simulink model "TestBench_DSD"  (R2021a)
settings: Solver=VariableStepAuto  StartTime=0.0  StopTime=0.05  FixedStep=1e-10  MaxStep=1e-4  RelTol=1e-3
PreLoadFcn:
  | clear;
  | dead_time= 5e-7;
  | T_sample = 1e-7;
  | f_pwm= 8e3;
  | f_el=200;
  | amplitude=0.1;
  | U_dc=800;
  | Iq_soll=200;
  | 
  | load('busdef.mat')
  | 
  | %**** Controller ****
  | L_filter = 70e-6;
  | R_losses = 1.74e-3;
  | PGain = L_filter*0.05*2*pi;
  | IGain = R_losses*0.05*2*pi;
  | 
  | %**** Deadtime Correction ****
  | Rds_on_module = 0.045/15;
  | 
  | %**** Filter ****
  | FilterQuality = 0.7071
InitFcn:
  | %%PGain = (L_filter*0.09*2*pi*f_pwm-R_losses)*0.45;
  | %%IGain = PGain*50/1.2; %% 25 = Period for ringing with too hight PGain
  | 
  | %%PGain = L_filter/(2*(1.5/f_pwm));
  | %%IGain  = PGain*R_losses/L_filter;
undefined symbols (not defined in the file): DiscIntNeverNeededParam, haltPwmSi, haltPwmSic, I_abc_sampled
libraries: nesl_utility x18, simulink x17, fl_lib x15, ee_lib x5, spsFirstOrderFilterLib x3, eeTransforms x2, cstextras x1, spsRMSLib x1, simulink_extras x1, spspowerguiLib x1
(part 2 of 3)

== system TestBench_DSD/Controller/Function-Call Subsystem4 ==
  function : TriggerPort  VariantControl=(inherit)
  Constant : Constant  Commented=on  Value=inf
  Constant1 : Constant  Commented=on
  Constant2 : Constant  Value=2
  Constant7 : Constant
  Data Store Read4 : DataStoreRead  DataStoreName=Inverter  IndexOptions=Index vector (dialog)  Indices=1  OutputSizes=1
  Data Store Write : DataStoreWrite  Commented=on  DataStoreName=Sic_PhU_ChB_On  IndexOptions=Index vector (dialog)  Indices=1  OutputSizes=1
  Data Store Write1 : DataStoreWrite  Commented=on  DataStoreName=Si_PhU_ChB_On  IndexOptions=Index vector (dialog)  Indices=1  OutputSizes=1
  Data Store Write2 : DataStoreWrite  DataStoreName=Inverter  IndexOptions=Index vector (dialog)  Indices=1  OutputSizes=1
  Data Store Write6 : DataStoreWrite  DataStoreName=haltPwmSi  DataStoreElements=haltPwmSi(2)  IndexOptions=Index vector (dialog)  Indices=1  OutputSizes=1
  MATLAB Function : MATLAB Function  TreatAsAtomicUnit=on
  wires:
  Constant/1 -> Data Store Write/1
  Constant1/1 -> Data Store Write1/1
  Constant7/1 -> Data Store Write6/1
  MATLAB Function/1(y) -> Data Store Write2/1
  Data Store Read4/1 -> MATLAB Function/2(devBus)
  Constant2/1 -> MATLAB Function/1(phase)

== system TestBench_DSD/Controller/Function-Call Subsystem5 ==
  function : TriggerPort  VariantControl=(inherit)
  Constant : Constant  Commented=on  Value=0
  Constant1 : Constant  Commented=on
  Constant2 : Constant  Commented=on  Value=0
  Constant3 : Constant  Commented=on  Value=-1
  Constant4 : Constant  Commented=on
  Constant5 : Constant  Commented=on
  Constant6 : Constant  Value=0
  Constant7 : Constant  Value=2
  Data Store Read4 : DataStoreRead  DataStoreName=Inverter  IndexOptions=Index vector (dialog)  Indices=1  OutputSizes=1
  Data Store Write : DataStoreWrite  Commented=on  DataStoreName=Sic_PhU_ChA_Off  IndexOptions=Index vector (dialog)  Indices=1  OutputSizes=1
  Data Store Write1 : DataStoreWrite  Commented=on  DataStoreName=Si_PhU_ChB_Off  IndexOptions=Index vector (dialog)  Indices=1  OutputSizes=1
  Data Store Write2 : DataStoreWrite  Commented=on  DataStoreName=Sic_PhU_ChA_On  IndexOptions=Index vector (dialog)  Indices=1  OutputSizes=1
  Data Store Write3 : DataStoreWrite  Commented=on  DataStoreName=Sic_PhU_ChB_Off  IndexOptions=Index vector (dialog)  Indices=1  OutputSizes=1
  Data Store Write4 : DataStoreWrite  Commented=on  DataStoreName=Si_PhU_ChA_Off  IndexOptions=Index vector (dialog)  Indices=1  OutputSizes=1
  Data Store Write5 : DataStoreWrite  Commented=on  DataStoreName=Si_PhU_ChA_On  IndexOptions=Index vector (dialog)  Indices=1  OutputSizes=1
  Data Store Write6 : DataStoreWrite  DataStoreName=Inverter  IndexOptions=Index vector (dialog)  Indices=1  OutputSizes=1
  Data Store Write7 : DataStoreWrite  DataStoreName=haltPwmSic  DataStoreElements=haltPwmSic(2)  IndexOptions=Index vector (dialog)  Indices=1  OutputSizes=1
  MATLAB Function : MATLAB Function  TreatAsAtomicUnit=on
  wires:
  Constant1/1 -> Data Store Write1/1
  Constant/1 -> Data Store Write/1
  Constant2/1 -> Data Store Write2/1
  Constant3/1 -> Data Store Write3/1
  Constant4/1 -> Data Store Write4/1
  Constant5/1 -> Data Store Write5/1
  Constant6/1 -> Data Store Write7/1
  MATLAB Function/1(y) -> Data Store Write6/1
  Data Store Read4/1 -> MATLAB Function/2(devBus)
  Constant7/1 -> MATLAB Function/1(phase)

== system TestBench_DSD/Controller/Function-Call Subsystem6 ==
  function : TriggerPort  VariantControl=(inherit)
  Constant : Constant  Commented=on
  Constant1 : Constant  Commented=on  Value=1e3
  Constant2 : Constant  Value=2
  Constant6 : Constant
  Data Store Read4 : DataStoreRead  DataStoreName=Inverter  IndexOptions=Index vector (dialog)  Indices=1  OutputSizes=1
  Data Store Write : DataStoreWrite  Commented=on  DataStoreName=Sic_PhU_ChB_On  IndexOptions=Index vector (dialog)  Indices=1  OutputSizes=1
  Data Store Write1 : DataStoreWrite  Commented=on  DataStoreName=Si_PhU_ChB_On  IndexOptions=Index vector (dialog)  Indices=1  OutputSizes=1
  Data Store Write2 : DataStoreWrite  DataStoreName=Inverter  IndexOptions=Index vector (dialog)  Indices=1  OutputSizes=1
  Data Store Write7 : DataStoreWrite  DataStoreName=haltPwmSic  DataStoreElements=haltPwmSic(2)  IndexOptions=Index vector (dialog)  Indices=1  OutputSizes=1
  MATLAB Function : MATLAB Function  TreatAsAtomicUnit=on
  wires:
  Constant/1 -> Data Store Write/1
  Constant1/1 -> Data Store Write1/1
  Constant6/1 -> Data Store Write7/1
  MATLAB Function/1(y) -> Data Store Write2/1
  Data Store Read4/1 -> MATLAB Function/2(devBus)
  Constant2/1 -> MATLAB Function/1(phase)

== system TestBench_DSD/Controller/Function-Call Subsystem7 ==
  function : TriggerPort  VariantControl=(inherit)
  Constant : Constant  Commented=on
  Constant1 : Constant  Commented=on  Value=-1
  Constant2 : Constant  Commented=on
  Constant3 : Constant  Commented=on
  Constant4 : Constant  Commented=on  Value=0
  Constant5 : Constant  Commented=on  Value=0
  Constant6 : Constant  Value=2
  Constant7 : Constant  Value=0
  Data Store Read4 : DataStoreRead  DataStoreName=Inverter  IndexOptions=Index vector (dialog)  Indices=1  OutputSizes=1
  Data Store Write : DataStoreWrite  Commented=on  DataStoreName=Sic_PhU_ChA_Off  IndexOptions=Index vector (dialog)  Indices=1  OutputSizes=1
  Data Store Write1 : DataStoreWrite  Commented=on  DataStoreName=Si_PhU_ChB_Off  IndexOptions=Index vector (dialog)  Indices=1  OutputSizes=1
  Data Store Write2 : DataStoreWrite  Commented=on  DataStoreName=Sic_PhU_ChA_On  IndexOptions=Index vector (dialog)  Indices=1  OutputSizes=1
  Data Store Write3 : DataStoreWrite  Commented=on  DataStoreName=Sic_PhU_ChB_Off  IndexOptions=Index vector (dialog)  Indices=1  OutputSizes=1
  Data Store Write4 : DataStoreWrite  Commented=on  DataStoreName=Si_PhU_ChA_Off  IndexOptions=Index vector (dialog)  Indices=1  OutputSizes=1
  Data Store Write5 : DataStoreWrite  Commented=on  DataStoreName=Si_PhU_ChA_On  IndexOptions=Index vector (dialog)  Indices=1  OutputSizes=1
  Data Store Write6 : DataStoreWrite  DataStoreName=haltPwmSi  DataStoreElements=haltPwmSi(2)  IndexOptions=Index vector (dialog)  Indices=1  OutputSizes=1
  Data Store Write7 : DataStoreWrite  DataStoreName=Inverter  IndexOptions=Index vector (dialog)  Indices=1  OutputSizes=1
  MATLAB Function : MATLAB Function  TreatAsAtomicUnit=on
  wires:
  Constant1/1 -> Data Store Write1/1
  Constant/1 -> Data Store Write/1
  Constant2/1 -> Data Store Write2/1
  Constant3/1 -> Data Store Write3/1
  Constant4/1 -> Data Store Write4/1
  Constant5/1 -> Data Store Write5/1
  Constant7/1 -> Data Store Write6/1
  Data Store Read4/1 -> MATLAB Function/2(devBus)
  MATLAB Function/1(y) -> Data Store Write7/1
  Constant6/1 -> MATLAB Function/1(phase)

== system TestBench_DSD/Controller/Function-Call Subsystem8 ==
  function : TriggerPort  VariantControl=(inherit)
  Constant : Constant  Commented=on  Value=inf
  Constant1 : Constant  Commented=on
  Constant2 : Constant  Value=3
  Constant7 : Constant
  Data Store Read4 : DataStoreRead  DataStoreName=Inverter  IndexOptions=Index vector (dialog)  Indices=1  OutputSizes=1
  Data Store Write : DataStoreWrite  Commented=on  DataStoreName=Sic_PhU_ChB_On  IndexOptions=Index vector (dialog)  Indices=1  OutputSizes=1
  Data Store Write1 : DataStoreWrite  Commented=on  DataStoreName=Si_PhU_ChB_On  IndexOptions=Index vector (dialog)  Indices=1  OutputSizes=1
  Data Store Write2 : DataStoreWrite  DataStoreName=Inverter  IndexOptions=Index vector (dialog)  Indices=1  OutputSizes=1
  Data Store Write6 : DataStoreWrite  DataStoreName=haltPwmSi  DataStoreElements=haltPwmSi(3)  IndexOptions=Index vector (dialog)  Indices=1  OutputSizes=1
  MATLAB Function : MATLAB Function  TreatAsAtomicUnit=on
  wires:
  Constant/1 -> Data Store Write/1
  Constant1/1 -> Data Store Write1/1
  Constant7/1 -> Data Store Write6/1
  MATLAB Function/1(y) -> Data Store Write2/1
  Data Store Read4/1 -> MATLAB Function/2(devBus)
  Constant2/1 -> MATLAB Function/1(phase)

== system TestBench_DSD/Controller/Function-Call Subsystem9 ==
  function : TriggerPort  VariantControl=(inherit)
  Constant : Constant  Commented=on  Value=0
  Constant1 : Constant  Commented=on
  Constant2 : Constant  Commented=on  Value=0
  Constant3 : Constant  Commented=on  Value=-1
  Constant4 : Constant  Commented=on
  Constant5 : Constant  Commented=on
  Constant6 : Constant  Value=0
  Constant7 : Constant  Value=3
  Data Store Read4 : DataStoreRead  DataStoreName=Inverter  IndexOptions=Index vector (dialog)  Indices=1  OutputSizes=1
  Data Store Write : DataStoreWrite  Commented=on  DataStoreName=Sic_PhU_ChA_Off  IndexOptions=Index vector (dialog)  Indices=1  OutputSizes=1
  Data Store Write1 : DataStoreWrite  Commented=on  DataStoreName=Si_PhU_ChB_Off  IndexOptions=Index vector (dialog)  Indices=1  OutputSizes=1
  Data Store Write2 : DataStoreWrite  Commented=on  DataStoreName=Sic_PhU_ChA_On  IndexOptions=Index vector (dialog)  Indices=1  OutputSizes=1
  Data Store Write3 : DataStoreWrite  Commented=on  DataStoreName=Sic_PhU_ChB_Off  IndexOptions=Index vector (dialog)  Indices=1  OutputSizes=1
  Data Store Write4 : DataStoreWrite  Commented=on  DataStoreName=Si_PhU_ChA_Off  IndexOptions=Index vector (dialog)  Indices=1  OutputSizes=1
  Data Store Write5 : DataStoreWrite  Commented=on  DataStoreName=Si_PhU_ChA_On  IndexOptions=Index vector (dialog)  Indices=1  OutputSizes=1
  Data Store Write6 : DataStoreWrite  DataStoreName=Inverter  IndexOptions=Index vector (dialog)  Indices=1  OutputSizes=1
  Data Store Write7 : DataStoreWrite  DataStoreName=haltPwmSic  DataStoreElements=haltPwmSic(3)  IndexOptions=Index vector (dialog)  Indices=1  OutputSizes=1
  MATLAB Function : MATLAB Function  TreatAsAtomicUnit=on
  wires:
  Constant1/1 -> Data Store Write1/1
  Constant/1 -> Data Store Write/1
  Constant2/1 -> Data Store Write2/1
  Constant3/1 -> Data Store Write3/1
  Constant4/1 -> Data Store Write4/1
  Constant5/1 -> Data Store Write5/1
  Constant6/1 -> Data Store Write7/1
  MATLAB Function/1(y) -> Data Store Write6/1
  Data Store Read4/1 -> MATLAB Function/2(devBus)
  Constant7/1 -> MATLAB Function/1(phase)

== system TestBench_DSD/Controller/Subsystem ==
  u : Inport
  cutoff frequency : Inport  Port=2
  Constant : Constant  Value=f_pwm
  MATLAB Function : cstextras/DiscreteFirstOrderSection/MATLAB Function  Tag=#GainSurfaceTarget_  SystemSampleTime=-1  VariantActivationTime=update diagram  Latency=0  AutoFrameSizeCalculation=off
      settings: SourceProductBaseCode=CT
  MATLAB Function1 : MATLAB Function  TreatAsAtomicUnit=on
  Product1 : Product
  Product4 : Product
  Sum : Sum  Inputs=|++
  Sum3 : Sum  Inputs=+|+
  Unit Delay : UnitDelay  SampleTime=-1  HasFrameUpgradeWarning=on
  y : Outport  VectorParamsAs1DForOutWhenUnconnected=off
  wires:
  u/1 -> Sum/1, Sum3/1
  Sum/1 -> Product1/2, Product4/2
  Product4/1 -> Sum3/2
  Sum3/1 -> Unit Delay/1
  cutoff frequency/1 -> MATLAB Function1/1(fc), MATLAB Function/1
  Unit Delay/1 -> Sum/2
  MATLAB Function/2 -> Product4/1
  MATLAB Function/1 -> Product1/1
  Product1/1 -> y/1
  MATLAB Function1/1(tau) -> MATLAB Function/2
  Constant/1 -> MATLAB Function1/2(fpwm)

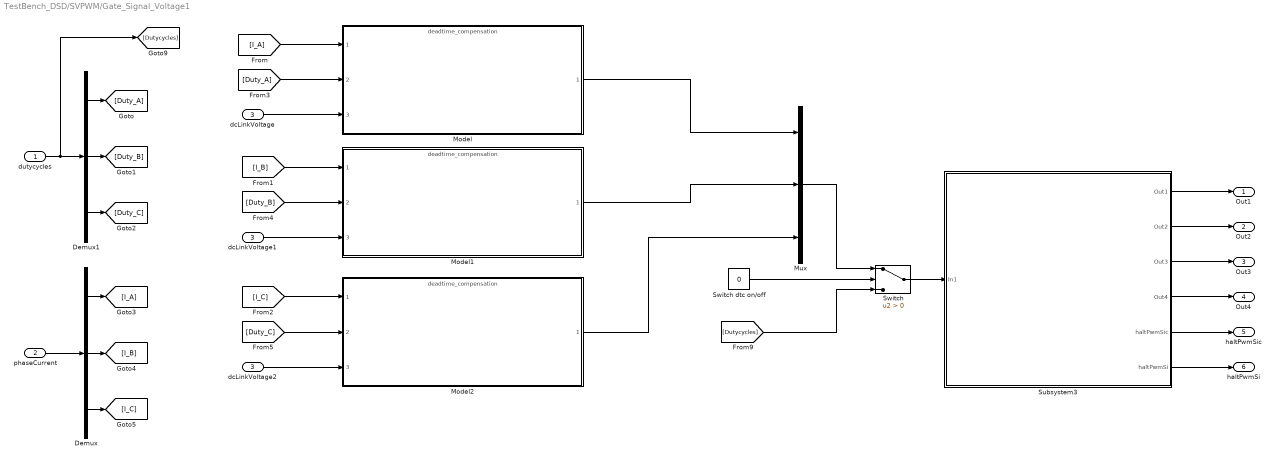
== system TestBench_DSD/SVPWM/Gate_Signal_Voltage1 ==
  dutycycles : Inport
  phaseCurrent : Inport  Port=2
  dcLinkVoltage : Inport  Port=3
  Demux : Demux  Outputs=3
  Demux1 : Demux  Outputs=3
  Model : ModelReference  ModelNameDialog=deadtime_compensation.slx  SimulationMode=Normal  ModelReferenceVersion=8.3
  Model1 : ModelReference  ModelNameDialog=deadtime_compensation.slx  SimulationMode=Normal  ModelReferenceVersion=8.3
  Model2 : ModelReference  ModelNameDialog=deadtime_compensation.slx  SimulationMode=Normal  ModelReferenceVersion=8.3
  Mux : Mux  Inputs=3
  Subsystem3 : Subsystem
  Switch : Switch  Criteria=u2 > Threshold
  Switch dtc on/off : Constant  Value=0
  dcLinkVoltage1 : InportShadow  Port=3
  dcLinkVoltage2 : InportShadow  Port=3
  Out1 : Outport
  Out2 : Outport  Port=2
  Out3 : Outport  Port=3
  Out4 : Outport  Port=4
  haltPwmSic : Outport  Port=5
  haltPwmSi : Outport  Port=6
  wires:
  phaseCurrent/1 -> Demux/1
  Demux1/1 -> [Duty_A]
  Demux1/2 -> [Duty_B]
  Demux1/3 -> [Duty_C]
  Demux/1 -> [I_A]
  Demux/2 -> [I_B]
  Demux/3 -> [I_C]
  [I_A] -> Model/1
  [Duty_A] -> Model/2
  Model/1 -> Mux/1
  [I_B] -> Model1/1
  [Duty_B] -> Model1/2
  Model1/1 -> Mux/2
  [Duty_C] -> Model2/2
  Switch dtc on/off/1 -> Switch/2
  [Dutycycles] -> Switch/3
  Mux/1 -> Switch/1
  dutycycles/1 -> Demux1/1, [Dutycycles]
  Model2/1 -> Mux/3
  Switch/1 -> Subsystem3/1(In1)
  Subsystem3/2(Out2) -> Out2/1
  Subsystem3/4(Out4) -> Out4/1
  Subsystem3/3(Out3) -> Out3/1
  Subsystem3/1(Out1) -> Out1/1
  Subsystem3/5(haltPwmSic) -> haltPwmSic/1
  Subsystem3/6(haltPwmSi) -> haltPwmSi/1
  [I_C] -> Model2/1
  dcLinkVoltage1/1 -> Model1/3
  dcLinkVoltage/1 -> Model/3
  dcLinkVoltage2/1 -> Model2/3

== system TestBench_DSD/SVPWM/SVPWM ==
  U_mag : Inport
  U_angle : Inport  Port=2
  Constant4 : Constant  Value=f_pwm
  Constant5 : Constant  Value=0
  Constant6 : Constant  Value=0
  Determine reference vector (U*) : Subsystem
  INFO : Subsystem
      mask Display: disp('?')
  SV Modulator Pattern #1 : Subsystem
  Sector Number : Outport  VectorParamsAs1DForOutWhenUnconnected=off
  Ta Tb T0 normalized : Outport  Port=2  VectorParamsAs1DForOutWhenUnconnected=off
  wires:
  SV Modulator Pattern #1/1(Sector Number) -> Sector Number/1
  SV Modulator Pattern #1/2(Ta Tb T0 normalized) -> Ta Tb T0 normalized/1
  U_angle/1 -> Determine reference vector (U*)/2(In2)
  Determine reference vector (U*)/2(alpha) -> SV Modulator Pattern #1/2(alpha)
  Constant6/1 -> Determine reference vector (U*)/5(Pha_Init)
  Determine reference vector (U*)/1(m) -> SV Modulator Pattern #1/1(m)
  Constant5/1 -> Determine reference vector (U*)/3(m_Int)
  Constant4/1 -> Determine reference vector (U*)/4(Freq_Int)
  U_mag/1 -> Determine reference vector (U*)/1(In1)

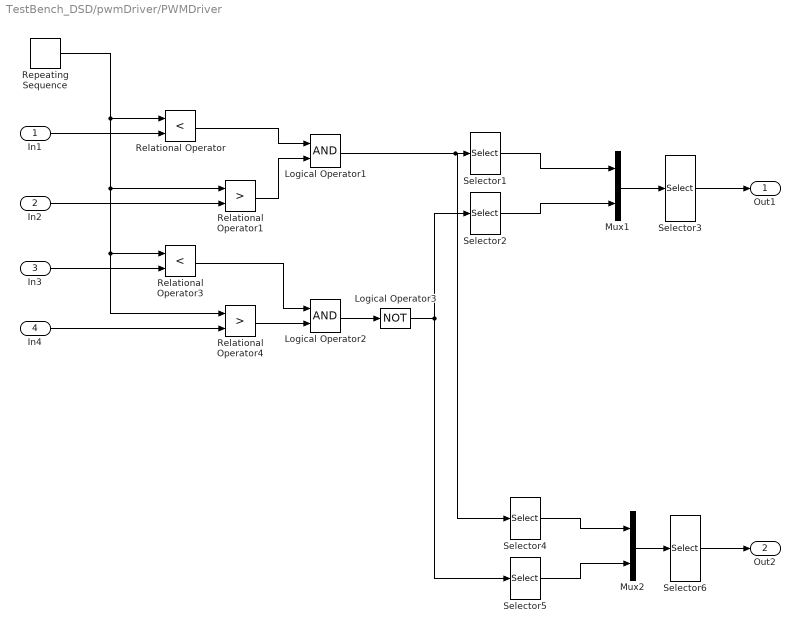
== system TestBench_DSD/pwmDriver/PWMDriver ==
  In1 : Inport
  In2 : Inport  Port=2
  In3 : Inport  Port=3
  In4 : Inport  Port=4
  Logical Operator1 : Logic  AllPortsSameDT=off  OutDataTypeStr=boolean
  Logical Operator2 : Logic  AllPortsSameDT=off  OutDataTypeStr=boolean
  Logical Operator3 : Logic  Operator=NOT  AllPortsSameDT=off  OutDataTypeStr=boolean
  Mux1 : Mux  Inputs=2
  Mux2 : Mux  Inputs=2
  Relational Operator : RelationalOperator  Operator=<  OutDataTypeStr=boolean  RndMeth=Simplest
  Relational Operator1 : RelationalOperator  Operator=>  OutDataTypeStr=boolean  RndMeth=Simplest
  Relational Operator3 : RelationalOperator  Operator=<  OutDataTypeStr=boolean  RndMeth=Simplest
  Relational Operator4 : RelationalOperator  Operator=>  OutDataTypeStr=boolean  RndMeth=Simplest
  Repeating Sequence : simulink/Sources/Repeating Sequence  rep_seq_t=[0 1/f_pwm]  rep_seq_y=[0 1/f_pwm]
  Selector1 : Selector  InputPortWidth=6  IndexOptions=Index vector (dialog)  Indices=[1 2 3]  OutputSizes=1
  Selector2 : Selector  InputPortWidth=6  IndexOptions=Index vector (dialog)  Indices=[1 2 3]  OutputSizes=1
  Selector3 : Selector  InputPortWidth=6  IndexOptions=Index vector (dialog)  Indices=[1 4 2 5 3 6]  OutputSizes=1
  Selector4 : Selector  InputPortWidth=6  IndexOptions=Index vector (dialog)  Indices=[4 5 6]  OutputSizes=1
  Selector5 : Selector  InputPortWidth=6  IndexOptions=Index vector (dialog)  Indices=[4 5 6]  OutputSizes=1
  Selector6 : Selector  InputPortWidth=6  IndexOptions=Index vector (dialog)  Indices=[1 4 2 5 3 6]  OutputSizes=1
  Out1 : Outport
  Out2 : Outport  Port=2
  wires:
  Repeating Sequence/1 -> Relational Operator/1, Relational Operator4/1, Relational Operator3/1, Relational Operator1/1
  Logical Operator1/1 -> Selector4/1, Selector1/1
  Mux1/1 -> Selector3/1
  Selector2/1 -> Mux1/2
  Mux2/1 -> Selector6/1
  Relational Operator3/1 -> Logical Operator2/1
  Logical Operator3/1 -> Selector5/1, Selector2/1
  Relational Operator4/1 -> Logical Operator2/2
  Logical Operator2/1 -> Logical Operator3/1
  In3/1 -> Relational Operator3/2
  Selector5/1 -> Mux2/2
  Relational Operator1/1 -> Logical Operator1/2
  Selector1/1 -> Mux1/1
  Relational Operator/1 -> Logical Operator1/1
  Selector4/1 -> Mux2/1
  Selector3/1 -> Out1/1
  Selector6/1 -> Out2/1
  In4/1 -> Relational Operator4/2
  In1/1 -> Relational Operator/2
  In2/1 -> Relational Operator1/2

== system TestBench_DSD/Controller/Discrete PI Controller Id/Clamping circuit ==
  preSat : Inport  DisableCoverage=on
  preIntegrator : Inport  DisableCoverage=on  Port=2
  AND : Logic  DisableCoverage=on
  Data Store Read1 : DataStoreRead  DataStoreName=dc_voltage_sampled  IndexOptions=Index vector (dialog)  Indices=1  OutputSizes=1
  Data Store Read5 : DataStoreRead  DataStoreName=dc_voltage_sampled  IndexOptions=Index vector (dialog)  Indices=1  OutputSizes=1
  DataTypeConv1 : DataTypeConversion  DisableCoverage=on  OutDataTypeStr=int8  SaturateOnIntegerOverflow=on  RndMeth=Zero  LockScale=on
  DataTypeConv2 : DataTypeConversion  DisableCoverage=on  OutDataTypeStr=int8
  Dead Zone Dynamic : simulink/Discontinuities/Dead Zone Dynamic
      settings: SourceProductBaseCode=SL
  Equal : RelationalOperator  DisableCoverage=on  Operator===  RndMeth=Nearest  InputSameDT=on
  Gain : Gain  Gain=-1
  NotEqual : RelationalOperator  DisableCoverage=on  Operator=~=  RndMeth=Nearest  InputSameDT=on
  SignDeltaU : Signum  DisableCoverage=on
  SignPreIntegrator : Signum  DisableCoverage=on
  ZeroGain : Gain  DisableCoverage=on  Gain=0  SaturateOnIntegerOverflow=on  OutDataTypeStr=Inherit: Same as input  ParamDataTypeStr=Inherit: Same as input
  Clamp : Outport  DisableCoverage=on  VectorParamsAs1DForOutWhenUnconnected=off
  wires:
  preSat/1 -> Dead Zone Dynamic/2, ZeroGain/1
  preIntegrator/1 -> SignPreIntegrator/1
  ZeroGain/1 -> NotEqual/1
  Dead Zone Dynamic/1 -> NotEqual/2, SignDeltaU/1
  SignDeltaU/1 -> DataTypeConv1/1
  DataTypeConv1/1 -> Equal/1
  SignPreIntegrator/1 -> DataTypeConv2/1
  DataTypeConv2/1 -> Equal/2
  NotEqual/1 -> AND/1
  Equal/1 -> AND/2
  AND/1 -> Clamp/1
  Data Store Read1/1 -> Gain/1
  Data Store Read5/1 -> Dead Zone Dynamic/1
  Gain/1 -> Dead Zone Dynamic/3

== system TestBench_DSD/Controller/Discrete PI Controller Iq/Clamping circuit ==
  preSat : Inport  DisableCoverage=on
  preIntegrator : Inport  DisableCoverage=on  Port=2
  AND : Logic  DisableCoverage=on
  Data Store Read1 : DataStoreRead  DataStoreName=dc_voltage_sampled  IndexOptions=Index vector (dialog)  Indices=1  OutputSizes=1
  Data Store Read5 : DataStoreRead  DataStoreName=dc_voltage_sampled  IndexOptions=Index vector (dialog)  Indices=1  OutputSizes=1
  DataTypeConv1 : DataTypeConversion  DisableCoverage=on  OutDataTypeStr=int8  SaturateOnIntegerOverflow=on  RndMeth=Zero  LockScale=on
  DataTypeConv2 : DataTypeConversion  DisableCoverage=on  OutDataTypeStr=int8
  Dead Zone Dynamic : simulink/Discontinuities/Dead Zone Dynamic
      settings: SourceProductBaseCode=SL
  Equal : RelationalOperator  DisableCoverage=on  Operator===  RndMeth=Nearest  InputSameDT=on
  Gain : Gain  Gain=-1
  NotEqual : RelationalOperator  DisableCoverage=on  Operator=~=  RndMeth=Nearest  InputSameDT=on
  SignDeltaU : Signum  DisableCoverage=on
  SignPreIntegrator : Signum  DisableCoverage=on
  ZeroGain : Gain  DisableCoverage=on  Gain=0  SaturateOnIntegerOverflow=on  OutDataTypeStr=Inherit: Same as input  ParamDataTypeStr=Inherit: Same as input
  Clamp : Outport  DisableCoverage=on  VectorParamsAs1DForOutWhenUnconnected=off
  wires:
  Gain/1 -> Dead Zone Dynamic/3
  Data Store Read5/1 -> Dead Zone Dynamic/1
  Data Store Read1/1 -> Gain/1
  AND/1 -> Clamp/1
  Equal/1 -> AND/2
  NotEqual/1 -> AND/1
  DataTypeConv2/1 -> Equal/2
  SignPreIntegrator/1 -> DataTypeConv2/1
  DataTypeConv1/1 -> Equal/1
  SignDeltaU/1 -> DataTypeConv1/1
  Dead Zone Dynamic/1 -> SignDeltaU/1, NotEqual/2
  ZeroGain/1 -> NotEqual/1
  preIntegrator/1 -> SignPreIntegrator/1
  preSat/1 -> ZeroGain/1, Dead Zone Dynamic/2

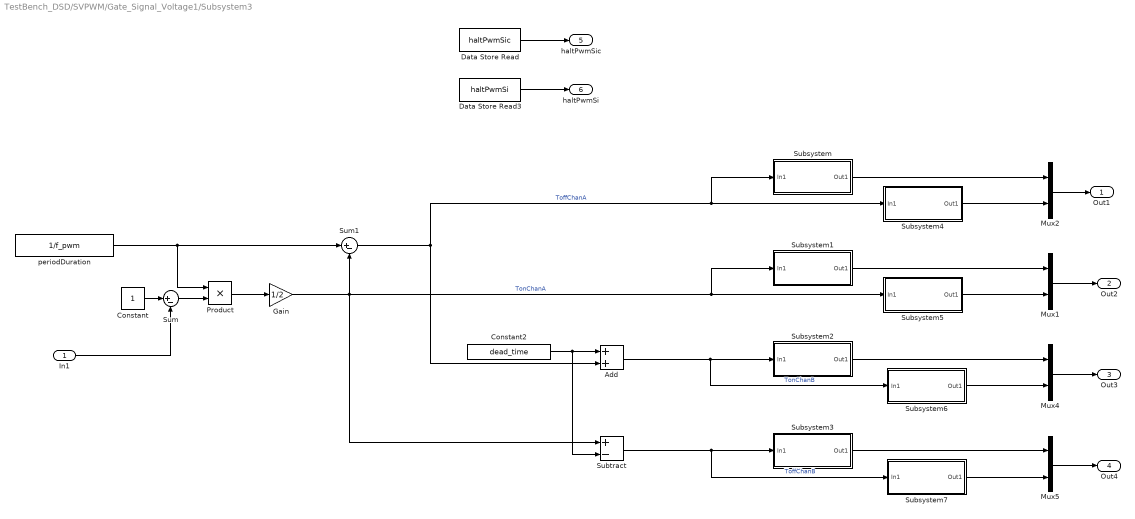
== system TestBench_DSD/SVPWM/Gate_Signal_Voltage1/Subsystem3 ==
  In1 : Inport
  Add : Sum
  Constant : Constant
  Constant2 : Constant  Value=dead_time
  Data Store Read : DataStoreRead  DataStoreName=haltPwmSic  IndexOptions=Index vector (dialog)  Indices=1  OutputSizes=1
  Data Store Read3 : DataStoreRead  DataStoreName=haltPwmSi  IndexOptions=Index vector (dialog)  Indices=1  OutputSizes=1
  Gain : Gain  Gain=1/2
  Mux{1..2,4..5} (4 alike) : Mux  Inputs=2
  Product : Product
  Subsystem : Subsystem
  Subsystem1 : Subsystem
  Subsystem2 : Subsystem
  Subsystem3 : Subsystem
  Subsystem4 : Subsystem
  Subsystem5 : Subsystem
  Subsystem6 : Subsystem
  Subsystem7 : Subsystem
  Subtract : Sum  Inputs=+-
  Sum : Sum  Inputs=|+-
  Sum1 : Sum  Inputs=|+-
  periodDuration : Constant  Value=1/f_pwm
  Out1 : Outport
  Out2 : Outport  Port=2
  Out3 : Outport  Port=3
  Out4 : Outport  Port=4
  haltPwmSic : Outport  Port=5
  haltPwmSi : Outport  Port=6
  wires:
  In1/1 -> Sum/2
  Constant2/1 -> Add/1, Subtract/2
  Sum1/1 -> Subsystem4/1(In1), Subsystem/1(In1), Add/2  "ToffChanA"
  periodDuration/1 -> Sum1/1, Product/1
  Gain/1 -> Subtract/1, Sum1/2, Subsystem5/1(In1), Subsystem1/1(In1)  "TonChanA"
  Constant/1 -> Sum/1
  Add/1 -> Subsystem2/1(In1), Subsystem6/1(In1)  "TonChanB"
  Product/1 -> Gain/1
  Mux2/1 -> Out1/1
  Subtract/1 -> Subsystem3/1(In1), Subsystem7/1(In1)  "ToffChanB"
  Mux4/1 -> Out3/1
  Sum/1 -> Product/2
  Mux5/1 -> Out4/1
  Mux1/1 -> Out2/1
  Subsystem/1(Out1) -> Mux2/1
  Subsystem1/1(Out1) -> Mux1/1
  Subsystem2/1(Out1) -> Mux4/1
  Subsystem3/1(Out1) -> Mux5/1
  Subsystem4/1(Out1) -> Mux2/2
  Subsystem5/1(Out1) -> Mux1/2
  Subsystem6/1(Out1) -> Mux4/2
  Subsystem7/1(Out1) -> Mux5/2
  Data Store Read/1 -> haltPwmSic/1
  Data Store Read3/1 -> haltPwmSi/1

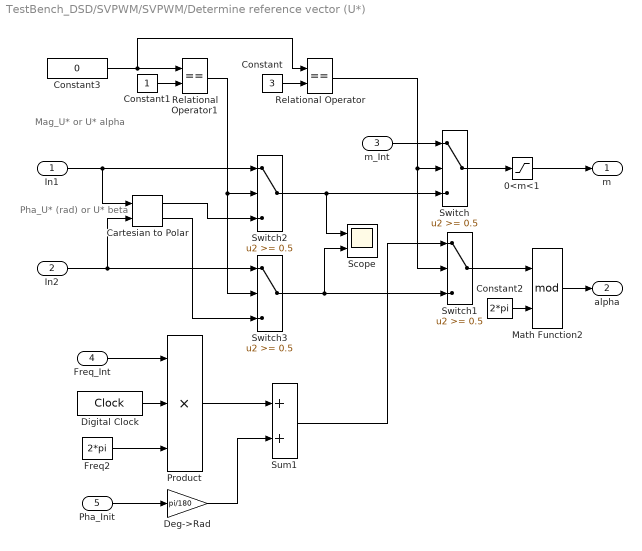
== system TestBench_DSD/SVPWM/SVPWM/Determine reference vector (U*) ==
  note: Pha_U* (rad)
      | or
      | U* beta
  note: Mag_U*
      | or
      | U* alpha
  In1 : Inport
  In2 : Inport  Port=2
  m_Int : Inport  Port=3
  Freq_Int : Inport  Port=4
  Pha_Init : Inport  Port=5
  "0<m<1 " : Saturate  UpperLimit=1  LowerLimit=0
  Cartesian to Polar : simulink_extras/Transformations/Cartesian to Polar
  Constant : Constant  Value=3
  Constant1 : Constant
  Constant2 : Constant  Value=2*pi
  Constant3 : Constant  Value=0
  Deg->Rad : Gain  Gain=pi/180  SaturateOnIntegerOverflow=on  OutDataTypeStr=Inherit: Same as input  ParamDataTypeStr=Inherit: Same as input
  Digital Clock : DigitalClock  SampleTime=-1
  Freq2 : Constant  Value=2*pi
  Math Function2 : Math  Operator=mod  SignedPower=on  SaturateOnIntegerOverflow=on
  Product : Product  Inputs=***  InputSameDT=on  SaturateOnIntegerOverflow=on  OutDataTypeStr=Inherit: Same as first input
  Relational Operator : RelationalOperator  Operator===  RndMeth=Nearest
  Relational Operator1 : RelationalOperator  Operator===  RndMeth=Nearest
  Scope : Scope  NumInputPorts=2
  Sum1 : Sum  InputSameDT=on  SaturateOnIntegerOverflow=on  OutDataTypeStr=Inherit: Same as first input
  Switch{,1..3} (4 alike) : Switch  Threshold=0.5  SaturateOnIntegerOverflow=on
  m : Outport  VectorParamsAs1DForOutWhenUnconnected=off
  alpha : Outport  Port=2  VectorParamsAs1DForOutWhenUnconnected=off
  wires:
  Digital Clock/1 -> Product/2
  Switch1/1 -> Math Function2/1
  Sum1/1 -> Switch1/1
  Math Function2/1 -> alpha/1
  Constant2/1 -> Math Function2/2
  Relational Operator1/1 -> Switch3/2, Switch2/2
  Cartesian to Polar/2 -> Switch3/3
  Cartesian to Polar/1 -> Switch2/3
  Switch2/1 -> Scope/1, Switch/3
  Constant3/1 -> Relational Operator/1, Relational Operator1/1
  Constant1/1 -> Relational Operator1/2
  Relational Operator/1 -> Switch/2, Switch1/2
  Constant/1 -> Relational Operator/2
  m_Int/1 -> Switch/1
  In2/1 -> Switch3/1, Cartesian to Polar/2
  In1/1 -> Switch2/1, Cartesian to Polar/1
  "0<m<1 "/1 -> m/1
  Switch/1 -> "0<m<1 "/1
  Freq2/1 -> Product/3
  Freq_Int/1 -> Product/1
  Deg->Rad/1 -> Sum1/2
  Pha_Init/1 -> Deg->Rad/1
  Product/1 -> Sum1/1
  Switch3/1 -> Scope/2, Switch1/3

== system TestBench_DSD/SVPWM/SVPWM/INFO ==
  note: Pattern #2:
      | With this pattern, identified as "Hardware-Determined" by Texas Instruments, there is always one PWM channel staying constant for the entire PWM period.
      |  So the number of switching times for this pattern is less than pattern #1. As a result, switching losses will be reduced with Pattern #2.
  note: Pattern #1:
      | With this pattern, identified as "Software-Determined" by Texas Instruments, each PWM channel switches twice per every PWM period.
  note: --------------------------------------------------------------------------------------------------------------------------------------------------------------------
  note: Reference: Application Report SPRA524
      | Space-Vector PWM with TMS320C24x Using H/W & S/W Determined Switching Patterns
      | Zhenyu Yu, Texas Instruments
  note: The objective of the SV PWM technique is to approximate the reference voltage vector (U*) instantaneously
      | by combination of the switching states corresponding to the basic space vectors.
  note: U7 = 1 1 1
  note: Q1 Q3 Q5
  note: --------------------------------------------------------
  note: Three-Phase VSC Diagram
  note: -
  note: +
  note: --------------------------------------------------------
  note: |
      | |
      | |
  note: ---Vc
  note: |
      | |
      | |
  note: |
      | |
      | |
      | |
      | |
      | |
  note: [Q6]
  note: [Q5]
  note: |
      | |
      | |
  note: ---Vb
  note: |
      | |
      | |
  note: |
      | |
      | |
      | |
      | |
      | |
  note: [Q4]
  note: [Q3]
  note: |
      | |
      | |
  note: ---Va
  note: |
      | |
      | |
  note: |
      | |
      | |
      | |
      | |
      | |
  note: [Q2]
  note: [Q1]
  note: Vdc
  note: [n] = Sector number
  note: [2]
  note: Basic Space Vectors and Switching States
  note: U4 = 0 1 1
  note: U5 = 0 0 1
  note: U6 = 1 0 1
  note: U0 = 0 0 0
  note: U3 = 0 1 0
  note: U2 = 1 1 0
  note: U1 = 1 0 0
  note: [6]
  note: [5]
  note: [4]
  note: [3]
  note: [1]
  note: 3                       2
      |       3                   2
      |         3               2
      |           3           2
      |             3       2
      |               3   2
      | 4 4 4 4 4 4 4 4 0 1 1 1 1 1 1 1 1
      |               5   6
      |             5       6
      |           5           6
      |         5               6
      |       5                   6
      |     5                       6
  note: Two symmetrical switching patterns have been implemented:

== system TestBench_DSD/SVPWM/SVPWM/SV Modulator Pattern #1 ==
  m : Inport
  alpha : Inport  Port=2
  "Compute time duration of switching states (Ta,Tb,To) " : Subsystem
  "Determine the sector of U* based on alpha (rad). Also, determine if the sector number is odd" : Subsystem
  INFO : Subsystem
      mask Display: disp('?')
  Sector Number : Outport  VectorParamsAs1DForOutWhenUnconnected=off
  Ta Tb T0 normalized : Outport  Port=2  VectorParamsAs1DForOutWhenUnconnected=off
  wires:
  m/1 -> "Compute time duration of switching states (Ta,Tb,To) "/2(m)
  alpha/1 -> "Compute time duration of switching states (Ta,Tb,To) "/1(alpha), "Determine the sector of U* based on alpha (rad). Also, determine if the sector number is odd"/1(alpha)
  "Compute time duration of switching states (Ta,Tb,To) "/1(Ta Tb T0 normalized) -> Ta Tb T0 normalized/1
  "Determine the sector of U* based on alpha (rad). Also, determine if the sector number is odd"/2(Odd_S) -> "Compute time duration of switching states (Ta,Tb,To) "/4(Odd_S)
  "Determine the sector of U* based on alpha (rad). Also, determine if the sector number is odd"/1(Sn) -> Sector Number/1, "Compute time duration of switching states (Ta,Tb,To) "/3(Sn)

== system TestBench_DSD/SVPWM/Gate_Signal_Voltage1/Subsystem3/Subsystem ==
  In1 : Inport
  Data Store Read2 : DataStoreRead  DataStoreName=Inverter  DataStoreElements=Inverter.V.Sic.ChA.TOn.enable  IndexOptions=Index vector (dialog)  Indices=1  OutputSizes=1
  Data Store Read4 : DataStoreRead  DataStoreName=Inverter  DataStoreElements=Inverter.U.Sic.ChA.TOn.enable  IndexOptions=Index vector (dialog)  Indices=1  OutputSizes=1
  Data Store Read5 : DataStoreRead  DataStoreName=Inverter  DataStoreElements=Inverter.W.Sic.ChA.TOn.enable  IndexOptions=Index vector (dialog)  Indices=1  OutputSizes=1
  Demux : Demux  Outputs=3
  Mux : Mux  Inputs=3
  Product : Product
  Product1 : Product
  Product2 : Product
  Out1 : Outport
  wires:
  In1/1 -> Demux/1
  Data Store Read4/1 -> Product/1
  Demux/1 -> Product/2
  Demux/2 -> Product1/2
  Demux/3 -> Product2/2
  Data Store Read5/1 -> Product2/1
  Data Store Read2/1 -> Product1/1
  Product1/1 -> Mux/2
  Mux/1 -> Out1/1
  Product2/1 -> Mux/3
  Product/1 -> Mux/1

== system TestBench_DSD/SVPWM/Gate_Signal_Voltage1/Subsystem3/Subsystem1 ==
  In1 : Inport
  Data Store Read : DataStoreRead  DataStoreName=Inverter  DataStoreElements=Inverter.U.Sic.ChA.TOff.enable  IndexOptions=Index vector (dialog)  Indices=1  OutputSizes=1
  Data Store Read1 : DataStoreRead  DataStoreName=Inverter  DataStoreElements=Inverter.V.Sic.ChA.TOff.enable  IndexOptions=Index vector (dialog)  Indices=1  OutputSizes=1
  Data Store Read3 : DataStoreRead  DataStoreName=Inverter  DataStoreElements=Inverter.W.Sic.ChA.TOff.enable  IndexOptions=Index vector (dialog)  Indices=1  OutputSizes=1
  Demux : Demux  Outputs=3
  Mux : Mux  Inputs=3
  Product : Product
  Product1 : Product
  Product2 : Product
  Out1 : Outport
  wires:
  Product/1 -> Mux/1
  Product2/1 -> Mux/3
  Mux/1 -> Out1/1
  Product1/1 -> Mux/2
  Data Store Read1/1 -> Product1/1
  Data Store Read3/1 -> Product2/1
  Demux/3 -> Product2/2
  Demux/2 -> Product1/2
  Demux/1 -> Product/2
  Data Store Read/1 -> Product/1
  In1/1 -> Demux/1

== system TestBench_DSD/SVPWM/Gate_Signal_Voltage1/Subsystem3/Subsystem2 ==
  In1 : Inport
  Data Store Read : DataStoreRead  DataStoreName=Inverter  DataStoreElements=Inverter.U.Sic.ChB.TOn.enable  IndexOptions=Index vector (dialog)  Indices=1  OutputSizes=1
  Data Store Read1 : DataStoreRead  DataStoreName=Inverter  DataStoreElements=Inverter.V.Sic.ChB.TOn.enable  IndexOptions=Index vector (dialog)  Indices=1  OutputSizes=1
  Data Store Read3 : DataStoreRead  DataStoreName=Inverter  DataStoreElements=Inverter.W.Sic.ChB.TOn.enable  IndexOptions=Index vector (dialog)  Indices=1  OutputSizes=1
  Demux : Demux  Outputs=3
  Mux : Mux  Inputs=3
  Product : Product
  Product1 : Product
  Product2 : Product
  Out1 : Outport
  wires:
  In1/1 -> Demux/1
  Data Store Read/1 -> Product/1
  Demux/1 -> Product/2
  Demux/2 -> Product1/2
  Demux/3 -> Product2/2
  Data Store Read3/1 -> Product2/1
  Data Store Read1/1 -> Product1/1
  Product1/1 -> Mux/2
  Mux/1 -> Out1/1
  Product2/1 -> Mux/3
  Product/1 -> Mux/1

== system TestBench_DSD/SVPWM/Gate_Signal_Voltage1/Subsystem3/Subsystem3 ==
  In1 : Inport
  Data Store Read : DataStoreRead  DataStoreName=Inverter  DataStoreElements=Inverter.U.Sic.ChB.TOff.enable  IndexOptions=Index vector (dialog)  Indices=1  OutputSizes=1
  Data Store Read1 : DataStoreRead  DataStoreName=Inverter  DataStoreElements=Inverter.V.Sic.ChB.TOff.enable  IndexOptions=Index vector (dialog)  Indices=1  OutputSizes=1
  Data Store Read3 : DataStoreRead  DataStoreName=Inverter  DataStoreElements=Inverter.W.Sic.ChB.TOff.enable  IndexOptions=Index vector (dialog)  Indices=1  OutputSizes=1
  Demux : Demux  Outputs=3
  Mux : Mux  Inputs=3
  Product : Product
  Product1 : Product
  Product2 : Product
  Out1 : Outport
  wires:
  Product/1 -> Mux/1
  Product2/1 -> Mux/3
  Mux/1 -> Out1/1
  Product1/1 -> Mux/2
  Data Store Read1/1 -> Product1/1
  Data Store Read3/1 -> Product2/1
  Demux/3 -> Product2/2
  Demux/2 -> Product1/2
  Demux/1 -> Product/2
  Data Store Read/1 -> Product/1
  In1/1 -> Demux/1

== system TestBench_DSD/SVPWM/Gate_Signal_Voltage1/Subsystem3/Subsystem4 ==
  In1 : Inport
  Data Store Read : DataStoreRead  DataStoreName=Inverter  DataStoreElements=Inverter.U.Si.ChA.TOn.enable  IndexOptions=Index vector (dialog)  Indices=1  OutputSizes=1
  Data Store Read1 : DataStoreRead  DataStoreName=Inverter  DataStoreElements=Inverter.V.Si.ChA.TOn.enable  IndexOptions=Index vector (dialog)  Indices=1  OutputSizes=1
  Data Store Read3 : DataStoreRead  DataStoreName=Inverter  DataStoreElements=Inverter.W.Si.ChA.TOn.enable  IndexOptions=Index vector (dialog)  Indices=1  OutputSizes=1
  Demux : Demux  Outputs=3
  Mux : Mux  Inputs=3
  Product : Product
  Product1 : Product
  Product2 : Product
  Out1 : Outport
  wires:
  Product/1 -> Mux/1
  Product2/1 -> Mux/3
  Mux/1 -> Out1/1
  Product1/1 -> Mux/2
  Data Store Read1/1 -> Product1/1
  Data Store Read3/1 -> Product2/1
  Demux/3 -> Product2/2
  Demux/2 -> Product1/2
  Demux/1 -> Product/2
  Data Store Read/1 -> Product/1
  In1/1 -> Demux/1

== system TestBench_DSD/SVPWM/Gate_Signal_Voltage1/Subsystem3/Subsystem5 ==
  In1 : Inport
  Data Store Read : DataStoreRead  DataStoreName=Inverter  DataStoreElements=Inverter.U.Si.ChA.TOff.enable  IndexOptions=Index vector (dialog)  Indices=1  OutputSizes=1
  Data Store Read1 : DataStoreRead  DataStoreName=Inverter  DataStoreElements=Inverter.V.Si.ChA.TOff.enable  IndexOptions=Index vector (dialog)  Indices=1  OutputSizes=1
  Data Store Read3 : DataStoreRead  DataStoreName=Inverter  DataStoreElements=Inverter.W.Si.ChA.TOff.enable  IndexOptions=Index vector (dialog)  Indices=1  OutputSizes=1
  Demux : Demux  Outputs=3
  Mux : Mux  Inputs=3
  Product : Product
  Product1 : Product
  Product2 : Product
  Out1 : Outport
  wires:
  In1/1 -> Demux/1
  Data Store Read/1 -> Product/1
  Demux/1 -> Product/2
  Demux/2 -> Product1/2
  Demux/3 -> Product2/2
  Data Store Read3/1 -> Product2/1
  Data Store Read1/1 -> Product1/1
  Product1/1 -> Mux/2
  Mux/1 -> Out1/1
  Product2/1 -> Mux/3
  Product/1 -> Mux/1

== system TestBench_DSD/SVPWM/Gate_Signal_Voltage1/Subsystem3/Subsystem6 ==
  In1 : Inport
  Data Store Read : DataStoreRead  DataStoreName=Inverter  DataStoreElements=Inverter.U.Si.ChB.TOn.enable  IndexOptions=Index vector (dialog)  Indices=1  OutputSizes=1
  Data Store Read1 : DataStoreRead  DataStoreName=Inverter  DataStoreElements=Inverter.V.Si.ChB.TOn.enable  IndexOptions=Index vector (dialog)  Indices=1  OutputSizes=1
  Data Store Read3 : DataStoreRead  DataStoreName=Inverter  DataStoreElements=Inverter.W.Si.ChB.TOn.enable  IndexOptions=Index vector (dialog)  Indices=1  OutputSizes=1
  Demux : Demux  Outputs=3
  Mux : Mux  Inputs=3
  Product : Product
  Product1 : Product
  Product2 : Product
  Out1 : Outport
  wires:
  Product/1 -> Mux/1
  Product2/1 -> Mux/3
  Mux/1 -> Out1/1
  Product1/1 -> Mux/2
  Data Store Read1/1 -> Product1/1
  Data Store Read3/1 -> Product2/1
  Demux/3 -> Product2/2
  Demux/2 -> Product1/2
  Demux/1 -> Product/2
  Data Store Read/1 -> Product/1
  In1/1 -> Demux/1

== system TestBench_DSD/SVPWM/Gate_Signal_Voltage1/Subsystem3/Subsystem7 ==
  In1 : Inport
  Data Store Read : DataStoreRead  DataStoreName=Inverter  DataStoreElements=Inverter.U.Si.ChB.TOff.enable  IndexOptions=Index vector (dialog)  Indices=1  OutputSizes=1
  Data Store Read1 : DataStoreRead  DataStoreName=Inverter  DataStoreElements=Inverter.V.Si.ChB.TOff.enable  IndexOptions=Index vector (dialog)  Indices=1  OutputSizes=1
  Data Store Read3 : DataStoreRead  DataStoreName=Inverter  DataStoreElements=Inverter.W.Si.ChB.TOff.enable  IndexOptions=Index vector (dialog)  Indices=1  OutputSizes=1
  Demux : Demux  Outputs=3
  Mux : Mux  Inputs=3
  Product : Product
  Product1 : Product
  Product2 : Product
  Out1 : Outport
  wires:
  In1/1 -> Demux/1
  Data Store Read/1 -> Product/1
  Demux/1 -> Product/2
  Demux/2 -> Product1/2
  Demux/3 -> Product2/2
  Data Store Read3/1 -> Product2/1
  Data Store Read1/1 -> Product1/1
  Product1/1 -> Mux/2
  Mux/1 -> Out1/1
  Product2/1 -> Mux/3
  Product/1 -> Mux/1

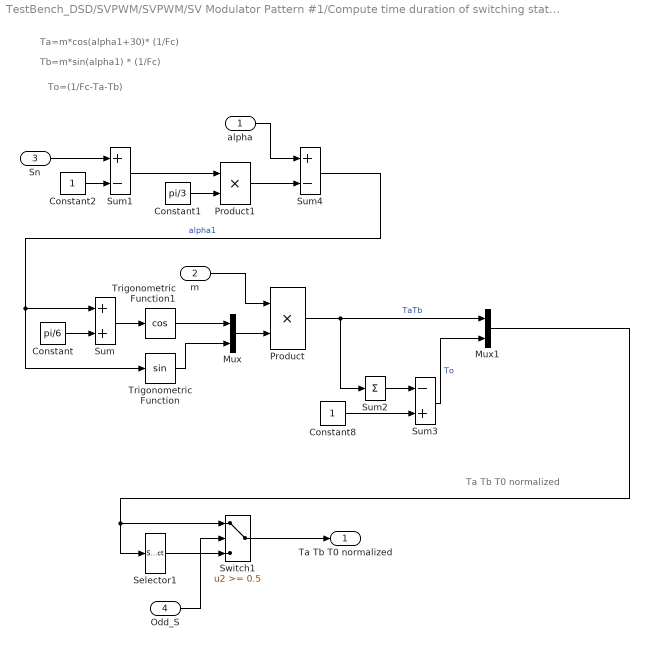
== system TestBench_DSD/SVPWM/SVPWM/SV Modulator Pattern #1/Compute time duration of switching states (Ta,Tb,To)  ==
  note: Ta Tb T0 normalized
  note: To=(1/Fc-Ta-Tb)
  note: Tb=m*sin(alpha1) * (1/Fc)
  note: Ta=m*cos(alpha1+30)* (1/Fc)
  alpha : Inport
  m : Inport  Port=2
  Sn : Inport  Port=3
  Odd_S : Inport  Port=4
  Constant : Constant  Value=pi/6
  Constant1 : Constant  Value=pi/3
  Constant2 : Constant
  Constant8 : Constant
  Mux : Mux  Inputs=2
  Mux1 : Mux  Inputs=2
  Product : Product  SaturateOnIntegerOverflow=on  OutDataTypeStr=Inherit: Same as first input
  Product1 : Product  SaturateOnIntegerOverflow=on  OutDataTypeStr=Inherit: Same as first input
  Selector1 : Selector  InputPortWidth=3  IndexOptions=Index vector (dialog)  Indices=[2 1 3]  OutputSizes=1
  Sum : Sum  SaturateOnIntegerOverflow=on
  Sum1 : Sum  Inputs=+-  SaturateOnIntegerOverflow=on
  Sum2 : Sum  Inputs=1  SaturateOnIntegerOverflow=on
  Sum3 : Sum  Inputs=-+  SaturateOnIntegerOverflow=on
  Sum4 : Sum  Inputs=+-  SaturateOnIntegerOverflow=on
  Switch1 : Switch  Threshold=0.5  SaturateOnIntegerOverflow=on
  Trigonometric Function : Trigonometry
  Trigonometric Function1 : Trigonometry  Operator=cos
  Ta Tb T0 normalized : Outport  VectorParamsAs1DForOutWhenUnconnected=off
  wires:
  Odd_S/1 -> Switch1/2
  Switch1/1 -> Ta Tb T0 normalized/1
  Selector1/1 -> Switch1/3
  Mux1/1 -> Selector1/1, Switch1/1
  Constant/1 -> Sum/2
  Sum4/1 -> Trigonometric Function/1, Sum/1  "alpha1"
  Sum3/1 -> Mux1/2  "To"
  Product/1 -> Sum2/1, Mux1/1  "TaTb"
  alpha/1 -> Sum4/1
  Product1/1 -> Sum4/2
  Constant2/1 -> Sum1/2
  Sn/1 -> Sum1/1
  Constant1/1 -> Product1/2
  Sum1/1 -> Product1/1
  Constant8/1 -> Sum3/2
  Sum2/1 -> Sum3/1
  Sum/1 -> Trigonometric Function1/1
  m/1 -> Product/1
  Mux/1 -> Product/2
  Trigonometric Function/1 -> Mux/2
  Trigonometric Function1/1 -> Mux/1

== system TestBench_DSD/SVPWM/SVPWM/SV Modulator Pattern #1/Determine the sector of U* based on alpha (rad). Also, determine if the sector number is odd ==
  alpha : Inport
  Constant1 : Constant  Value=2
  Look-Up Table : Lookup  InputValues=[0:pi/3:5*pi/3]  Table=[1:6]  LookUpMeth=Interpolation-Use End Values  SaturateOnIntegerOverflow=on
  Math Function1 : Math  Operator=mod  SignedPower=on  SaturateOnIntegerOverflow=on
  Rounding Function : Rounding
  Sn : Outport  VectorParamsAs1DForOutWhenUnconnected=off
  Odd_S : Outport  Port=2  VectorParamsAs1DForOutWhenUnconnected=off
  wires:
  alpha/1 -> Look-Up Table/1
  Math Function1/1 -> Odd_S/1
  Constant1/1 -> Math Function1/2
  Rounding Function/1 -> Sn/1, Math Function1/1
  Look-Up Table/1 -> Rounding Function/1

== system TestBench_DSD/SVPWM/SVPWM/SV Modulator Pattern #1/INFO ==
  note: Interval 7
  note: Interval 6
  note: Interval 5
  note: Interval 4
  note: Interval 3
  note: Interval 2
  note: Interval 1
  note: zero
      | space vector
      | (Q1 Q3 Q5 =0)
  note: 1st basic
      | space vector
  note: 2nd basic
      | space vector
  note: zero
      | space vector
      | (Q1 Q3 Q5 =1)
  note: zero
      | space vector
      | (Q1 Q3 Q5 =0)
  note: 2nd basic
      | space vector
  note: 1st basic
      | space vector
  note: Pattern #1 implements the following symmetrical switching pattern:
      | total duration = 1 PWM period (Tpwm = 1/Fc)
  note: |
      | |
      | |
      | |
      | |
      | |
      | |
      | |
      | |
      | |
  note: |
      | |
      | |
      | |
      | |
      | |
      | |
      | |
      | |
      | |
  note: |
      | |
      | |
      | |
      | |
      | |
      | |
      | |
      | |
      | |
  note: |
      | |
      | |
      | |
      | |
      | |
      | |
      | |
      | |
      | |
  note: |
      | |
      | |
      | |
      | |
      | |
      | |
      | |
      | |
      | |
  note: |
      | |
      | |
      | |
      | |
      | |
      | |
      | |
      | |
      | |
  note: Ta/2
  note: To/4
  note: Tb/2
  note: To/2
  note: Tb/2
  note: Ta/2
  note: To/4
  note: Ta=m*cos(alpha+30)* (1/Fc)
  note: Tb=m*sin(alpha) * (1/Fc)
  note: To=(1/Fc-Ta-Tb)
  note: where:
      | Fc = Chopping frequency
      | m = modulation index
      | alpha = angle between reference vector U* and
      | 1st basic space vector

== matlab function TestBench_DSD/Controller/Function-Call Subsystem9/MATLAB Function ==
  data: phase input; y output Bus: Device; devBus input Bus: Device
function y = fcn(phase,devBus)

switch phase 

    case 1
        
        devBus.U.Sic.ChA.TOn.enable = 0;
        devBus.U.Sic.ChA.TOff.enable = 0;

        devBus.U.Sic.ChB.TOff.enable = -1;

        devBus.U.Si.ChA.TOn.enable = 1;
        devBus.U.Si.ChA.TOff.enable = 1;

        devBus.U.Si.ChB.TOff.enable  = 1;

    case 2

        devBus.V.Sic.ChA.TOn.enable = 0;
        devBus.V.Sic.ChA.TOff.enable = 0;

        devBus.V.Sic.ChB.TOff.enable = -1;

        devBus.V.Si.ChA.TOn.enable = 1;
        devBus.V.Si.ChA.TOff.enable = 1;

        devBus.V.Si.ChB.TOff.enable  = 1;

    case 3

        devBus.W.Sic.ChA.TOn.enable = 0;
        devBus.W.Sic.ChA.TOff.enable = 0;

        devBus.W.Sic.ChB.TOff.enable = -1;

        devBus.W.Si.ChA.TOn.enable = 1;
        devBus.W.Si.ChA.TOff.enable = 1;

        devBus.W.Si.ChB.TOff.enable  = 1;
    
    otherwise
        error('No phase specified');

end

y = devBus;

== matlab function TestBench_DSD/Controller/Subsystem/MATLAB Function1 ==
  data: fc input; fpwm input; tau output
function tau = fcn(fc, fpwm)

delta_t = 1/fpwm;
tau     = 1/(2*pi*fc);
alpha   = delta_t / (tau+delta_t);
tau     = -(delta_t/(log(alpha)));

end

== matlab function TestBench_DSD/Controller/Function-Call Subsystem2/MATLAB Function ==
  data: phase input; y output Bus: Device; devBus input Bus: Device
function y = fcn(phase,devBus)

switch phase 

    case 1

        devBus.U.Sic.ChB.TOn.enable = 1;
        devBus.U.Si.ChB.TOn.enable  = inf;

    case 2

        devBus.V.Sic.ChB.TOn.enable = 1;
        devBus.V.Si.ChB.TOn.enable  = inf;

    case 3

        devBus.W.Sic.ChB.TOn.enable = 1;
        devBus.W.Si.ChB.TOn.enable  = inf;
    
    otherwise
        error('No phase specified');

end

y = devBus;

== matlab function TestBench_DSD/Controller/Function-Call Subsystem1/MATLAB Function ==
  data: phase input; y output Bus: Device; devBus input Bus: Device
function y = fcn(phase,devBus)

switch phase 

    case 1
        
        devBus.U.Sic.ChA.TOn.enable = 0;
        devBus.U.Sic.ChA.TOff.enable = 0;

        devBus.U.Sic.ChB.TOff.enable = -1;

        devBus.U.Si.ChA.TOn.enable = 1;
        devBus.U.Si.ChA.TOff.enable = 1;

        devBus.U.Si.ChB.TOff.enable  = 1;

    case 2

        devBus.V.Sic.ChA.TOn.enable = 0;
        devBus.V.Sic.ChA.TOff.enable = 0;

        devBus.V.Sic.ChB.TOff.enable = -1;

        devBus.V.Si.ChA.TOn.enable = 1;
        devBus.V.Si.ChA.TOff.enable = 1;

        devBus.V.Si.ChB.TOff.enable  = 1;

    case 3

        devBus.W.Sic.ChA.TOn.enable = 0;
        devBus.W.Sic.ChA.TOff.enable = 0;

        devBus.W.Sic.ChB.TOff.enable = -1;

        devBus.W.Si.ChA.TOn.enable = 1;
        devBus.W.Si.ChA.TOff.enable = 1;

        devBus.W.Si.ChB.TOff.enable  = 1;
    
    otherwise
        error('No phase specified');

end

y = devBus;

== matlab function TestBench_DSD/Controller/Function-Call Subsystem3/MATLAB Function ==
  data: phase input; y output Bus: Device; devBus input Bus: Device
function y = fcn(phase,devBus)

switch phase 

    case 1
        
        devBus.U.Sic.ChA.TOn.enable = 1;
        devBus.U.Sic.ChA.TOff.enable = 1;

        devBus.U.Sic.ChB.TOff.enable = 1;

        devBus.U.Si.ChA.TOn.enable = 0;
        devBus.U.Si.ChA.TOff.enable = 0;

        devBus.U.Si.ChB.TOff.enable  = -1;

    case 2

        devBus.V.Sic.ChA.TOn.enable = 1;
        devBus.V.Sic.ChA.TOff.enable = 1;

        devBus.V.Sic.ChB.TOff.enable = 1;

        devBus.V.Si.ChA.TOn.enable = 0;
        devBus.V.Si.ChA.TOff.enable = 0;

        devBus.V.Si.ChB.TOff.enable  = -1;

    case 3

        devBus.W.Sic.ChA.TOn.enable = 1;
        devBus.W.Sic.ChA.TOff.enable = 1;

        devBus.W.Sic.ChB.TOff.enable = 1;

        devBus.W.Si.ChA.TOn.enable = 0;
        devBus.W.Si.ChA.TOff.enable = 0;

        devBus.W.Si.ChB.TOff.enable  = -1;
    
    otherwise
        error('No phase specified');

end

y = devBus;

== matlab function TestBench_DSD/Controller/Function-Call Subsystem4/MATLAB Function ==
  data: phase input; y output Bus: Device; devBus input Bus: Device
function y = fcn(phase,devBus)

switch phase 

    case 1

        devBus.U.Sic.ChB.TOn.enable = inf;
        devBus.U.Si.ChB.TOn.enable  = 1;

    case 2

        devBus.V.Sic.ChB.TOn.enable = inf;
        devBus.V.Si.ChB.TOn.enable  = 1;

    case 3

        devBus.W.Sic.ChB.TOn.enable = inf;
        devBus.W.Si.ChB.TOn.enable  = 1;
    
    otherwise
        error('No phase specified');

end

y = devBus;

== matlab function TestBench_DSD/Controller/Function-Call Subsystem5/MATLAB Function ==
  data: phase input; y output Bus: Device; devBus input Bus: Device
function y = fcn(phase,devBus)

switch phase 

    case 1
        
        devBus.U.Sic.ChA.TOn.enable = 0;
        devBus.U.Sic.ChA.TOff.enable = 0;

        devBus.U.Sic.ChB.TOff.enable = -1;

        devBus.U.Si.ChA.TOn.enable = 1;
        devBus.U.Si.ChA.TOff.enable = 1;

        devBus.U.Si.ChB.TOff.enable  = 1;

    case 2

        devBus.V.Sic.ChA.TOn.enable = 0;
        devBus.V.Sic.ChA.TOff.enable = 0;

        devBus.V.Sic.ChB.TOff.enable = -1;

        devBus.V.Si.ChA.TOn.enable = 1;
        devBus.V.Si.ChA.TOff.enable = 1;

        devBus.V.Si.ChB.TOff.enable  = 1;

    case 3

        devBus.W.Sic.ChA.TOn.enable = 0;
        devBus.W.Sic.ChA.TOff.enable = 0;

        devBus.W.Sic.ChB.TOff.enable = -1;

        devBus.W.Si.ChA.TOn.enable = 1;
        devBus.W.Si.ChA.TOff.enable = 1;

        devBus.W.Si.ChB.TOff.enable  = 1;
    
    otherwise
        error('No phase specified');

end

y = devBus;

== matlab function TestBench_DSD/Controller/Function-Call Subsystem6/MATLAB Function ==
  data: phase input; y output Bus: Device; devBus input Bus: Device
function y = fcn(phase,devBus)

switch phase 

    case 1

        devBus.U.Sic.ChB.TOn.enable = 1;
        devBus.U.Si.ChB.TOn.enable  = inf;

    case 2

        devBus.V.Sic.ChB.TOn.enable = 1;
        devBus.V.Si.ChB.TOn.enable  = inf;

    case 3

        devBus.W.Sic.ChB.TOn.enable = 1;
        devBus.W.Si.ChB.TOn.enable  = inf;
    
    otherwise
        error('No phase specified');

end

y = devBus;

== matlab function TestBench_DSD/Controller/Function-Call Subsystem7/MATLAB Function ==
  data: phase input; y output Bus: Device; devBus input Bus: Device
function y = fcn(phase,devBus)

switch phase 

    case 1
        
        devBus.U.Sic.ChA.TOn.enable = 1;
        devBus.U.Sic.ChA.TOff.enable = 1;

        devBus.U.Sic.ChB.TOff.enable = 1;

        devBus.U.Si.ChA.TOn.enable = 0;
        devBus.U.Si.ChA.TOff.enable = 0;

        devBus.U.Si.ChB.TOff.enable  = -1;

    case 2

        devBus.V.Sic.ChA.TOn.enable = 1;
        devBus.V.Sic.ChA.TOff.enable = 1;

        devBus.V.Sic.ChB.TOff.enable = 1;

        devBus.V.Si.ChA.TOn.enable = 0;
        devBus.V.Si.ChA.TOff.enable = 0;

        devBus.V.Si.ChB.TOff.enable  = -1;

    case 3

        devBus.W.Sic.ChA.TOn.enable = 1;
        devBus.W.Sic.ChA.TOff.enable = 1;

        devBus.W.Sic.ChB.TOff.enable = 1;

        devBus.W.Si.ChA.TOn.enable = 0;
        devBus.W.Si.ChA.TOff.enable = 0;

        devBus.W.Si.ChB.TOff.enable  = -1;
    
    otherwise
        error('No phase specified');

end

y = devBus;

== matlab function TestBench_DSD/Controller/Function-Call Subsystem/MATLAB Function ==
  data: phase input; y output Bus: Device; devBus input Bus: Device
function y = fcn(phase,devBus)

switch phase 

    case 1

        devBus.U.Sic.ChB.TOn.enable = inf;
        devBus.U.Si.ChB.TOn.enable  = 1;

    case 2

        devBus.V.Sic.ChB.TOn.enable = inf;
        devBus.V.Si.ChB.TOn.enable  = 1;

    case 3

        devBus.W.Sic.ChB.TOn.enable = inf;
        devBus.W.Si.ChB.TOn.enable  = 1;
    
    otherwise
        error('No phase specified');

end

y = devBus;

== matlab function TestBench_DSD/Controller/Function-Call Subsystem10/MATLAB Function ==
  data: phase input; y output Bus: Device; devBus input Bus: Device
function y = fcn(phase,devBus)

switch phase 

    case 1

        devBus.U.Sic.ChB.TOn.enable = 1;
        devBus.U.Si.ChB.TOn.enable  = inf;

    case 2

        devBus.V.Sic.ChB.TOn.enable = 1;
        devBus.V.Si.ChB.TOn.enable  = inf;

    case 3

        devBus.W.Sic.ChB.TOn.enable = 1;
        devBus.W.Si.ChB.TOn.enable  = inf;
    
    otherwise
        error('No phase specified');

end

y = devBus;

== matlab function TestBench_DSD/Controller/Function-Call Subsystem11/MATLAB Function ==
  data: phase input; y output Bus: Device; devBus input Bus: Device
function y = fcn(phase,devBus)

switch phase 

    case 1
        
        devBus.U.Sic.ChA.TOn.enable = 1;
        devBus.U.Sic.ChA.TOff.enable = 1;

        devBus.U.Sic.ChB.TOff.enable = 1;

        devBus.U.Si.ChA.TOn.enable = 0;
        devBus.U.Si.ChA.TOff.enable = 0;

        devBus.U.Si.ChB.TOff.enable  = -1;

    case 2

        devBus.V.Sic.ChA.TOn.enable = 1;
        devBus.V.Sic.ChA.TOff.enable = 1;

        devBus.V.Sic.ChB.TOff.enable = 1;

        devBus.V.Si.ChA.TOn.enable = 0;
        devBus.V.Si.ChA.TOff.enable = 0;

        devBus.V.Si.ChB.TOff.enable  = -1;

    case 3

        devBus.W.Sic.ChA.TOn.enable = 1;
        devBus.W.Sic.ChA.TOff.enable = 1;

        devBus.W.Sic.ChB.TOff.enable = 1;

        devBus.W.Si.ChA.TOn.enable = 0;
        devBus.W.Si.ChA.TOff.enable = 0;

        devBus.W.Si.ChB.TOff.enable  = -1;
    
    otherwise
        error('No phase specified');

end

y = devBus;
